simulink model "untitled"  (R2019b)
settings: Solver=VariableStepAuto  StartTime=0.0  StopTime=1  RelTol=1e-3
libraries: powerlib_meascontrol x1, powerlib x1
settings Model: Creator=付  LastModifiedBy=付

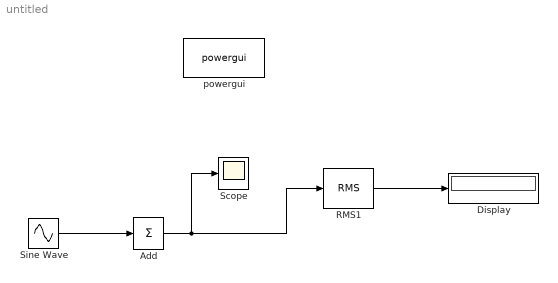
== system untitled ==
  Add : Sum  Inputs=1
  Display : Display
  RMS1 : powerlib_meascontrol/Measurements/RMS  TrueRMS=on  Freq=1  RMSInit=120  Ts=0
      settings: SourceProductName=Simscape Electrical
  Scope : Scope
  Sine Wave : Sin  Amplitude=0.75  Bias=3.75  Frequency=1*2*pi  SampleTime=0
  powergui : powerlib/powergui  Priority=1  SimulationMode=Continuous  SampleTime=50e-6  frequency=60  Iterations=50  frequencyindice=6  Pbase=100e6  ErrMax=1e-4  UnitsV=kV  UnitsW=MW  buscounter=0  FunctionMessages=off  echomessages=off  EnableUseOfTLC=off  CurrentSourceSwitches=off  DisableSnubberDevices=off  DisableRonSwitches=off  DisableVfSwitches=off  DisplayEquations=off  AutomaticDiscreteSolvers=off  SolverType=Tustin/Backward Euler (TBE)  Interpol=off  ExternalGateDelay=off  methode=off  Ts=100  x0status=blocks  SPID=on  SwTol=0  HookPort=off  NonlinearTolerance=1e-4  nMaxIteration=100  ContinueOnMaxIteration=off  RestoreLinks=warning  ResistiveCurrentMeasurement=off  Frange=[0:2:500]  Ylog=off  Xlog=on  ShowGrid=off  save=off  variable=ZData  structure=0  ZoomFFT=off  StartTime=0.0  cycles=1  DisplayStyle=1  fundamental=60  FreqAxis=off  MaxFrequency=1000  frequencyindicesteady=1  RmsSteady=1  display=off
      settings: SourceProductName=Simscape Electrical
  wires:
  RMS1/1 -> Display/1
  Sine Wave/1 -> Add/1
  Add/1 -> Scope/1, RMS1/1
